simulink model "Train20"  (R2020b)
settings: Solver=VariableStepAuto  StartTime=0.0  StopTime=10.0  RelTol=1e-3
model workspace (MAT data in the model file):
  M_1 = 1
  M_10 = 1
  M_11 = 1
  M_12 = 1
  M_13 = 1
  M_14 = 1
  M_15 = 1
  M_16 = 1
  M_17 = 1
  M_18 = 1
  M_19 = 1
  M_2 = 1
  M_20 = 1
  M_3 = 1
  M_4 = 1
  M_5 = 1
  M_6 = 1
  M_7 = 1
  M_8 = 1
  M_9 = 1
  X0_10 = 1
  X0_11 = 1
  X0_12 = 1
  X0_13 = 1
  X0_14 = 1
  X0_15 = 1
  X0_16 = 1
  X0_17 = 1
  X0_18 = 1
  X0_19 = 1
  X0_2 = 1
  X0_20 = 1
  X0_3 = 1
  X0_4 = 1
  X0_5 = 1
  X0_6 = 1
  X0_7 = 1
  X0_8 = 1
  X0_9 = 1
  c = 8
  h = 1
  hs = 1
  k = 0.1
settings Model: Creator=zhenya  LastModifiedBy=zhenya

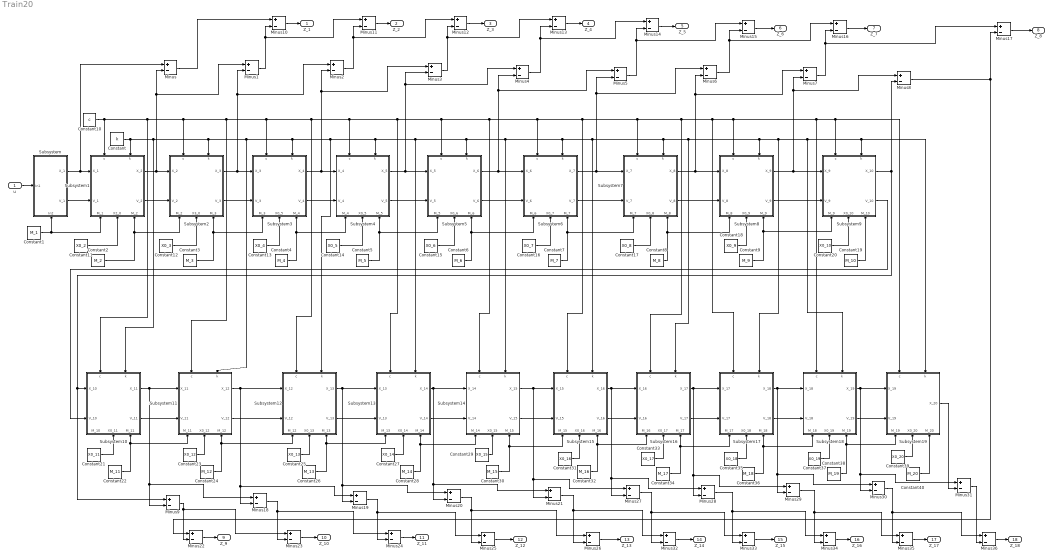
== system Train20 ==
  u : Inport
  Constant : Constant  Value=k
  Constant1 : Constant  Value=M_1
  Constant10 : Constant  Value=c
  Constant11 : Constant  Value=X0_2
  Constant12 : Constant  Value=X0_3
  Constant13 : Constant  Value=X0_4
  Constant14 : Constant  Value=X0_5
  Constant15 : Constant  Value=X0_6
  Constant16 : Constant  Value=X0_7
  Constant17 : Constant  Value=X0_8
  Constant18 : Constant  Value=X0_9
  Constant19 : Constant  Value=M_10
  Constant2 : Constant  Value=M_2
  Constant20 : Constant  Value=X0_10
  Constant21 : Constant  Value=X0_11
  Constant22 : Constant  Value=M_11
  Constant23 : Constant  Value=X0_12
  Constant24 : Constant  Value=M_12
  Constant25 : Constant  Value=X0_13
  Constant26 : Constant  Value=M_13
  Constant27 : Constant  Value=X0_14
  Constant28 : Constant  Value=M_14
  Constant29 : Constant  Value=X0_15
  Constant3 : Constant  Value=M_3
  Constant30 : Constant  Value=M_15
  Constant31 : Constant  Value=X0_16
  Constant32 : Constant  Value=M_16
  Constant33 : Constant  Value=X0_17
  Constant34 : Constant  Value=M_17
  Constant35 : Constant  Value=X0_18
  Constant36 : Constant  Value=M_18
  Constant37 : Constant  Value=X0_19
  Constant38 : Constant  Value=M_19
  Constant39 : Constant  Value=X0_20
  Constant4 : Constant  Value=M_4
  Constant40 : Constant  Value=M_20
  Constant5 : Constant  Value=M_5
  Constant6 : Constant  Value=M_6
  Constant7 : Constant  Value=M_7
  Constant8 : Constant  Value=M_8
  Constant9 : Constant  Value=M_9
  Minus{,1..36} (37 alike) : Sum  Inputs=+-
  Subsystem : Subsystem
      settings: PortSchema="{\"entries\":[{\"content\":{\"sides\":[{\"content\":{\"connectorIds\":[\"In1\"]},\"type\":\"ConnectorPlacement.EquallySpacedRectSide\",\"uuid\":\"34ca8425-fccb-4da0-be07-954015c86f74\"},{\"content\":{\"connectorIds\":[\"Out1\",\"Out2\"],\"side\":\"RIGHT\"},\"type\":\"ConnectorPlacement.EquallySpacedRectSide\",\"uuid\":\"a4a70c44-d99b-4f2f-bcd7-1dd85156dc1f\"},{\"content\":{\"connectorIds\":[],\"side\":\"TOP\"},\"type\":\"ConnectorPlacement.EquallySpacedRectSide\",\"uuid\":\"14968497-3b66-4f95-885e-db1a1d92cb6f\"},{\"content\":{\"connectorIds\":[\"In2\"],\"side\":\"BOTTOM\"},\"type\":\"ConnectorPlacement.EquallySpacedRectSide\",\"uuid\":\"7000d41a-f478-4b38-bf4d-e27f7f915c37\"},{\"content\":{\"connectorIds\":[],\"side\":\"HIDDEN\"},\"type\":\"ConnectorPlacement.EquallySpacedRectSide\",\"uuid\":\"79f1d2cd-3fc8-42f6-ae8b-07eaf6f97827\"}]},\"type\":\"ConnectorPlacement.EquallySpacedConnector\",\"uuid\":\"0ff0aa4c-6fa5-4dba-bb7c-396d165f33e0\"}],\"packageUris\":[\"http://schema.mathworks.com/mf0/Connector/R2020b\"],\"version\":\"1.0\"}"
  Subsystem1 : Subsystem
      settings: PortSchema="{\"entries\":[{\"content\":{\"sides\":[{\"content\":{\"connectorIds\":[\"In1\",\"In2\"]},\"type\":\"ConnectorPlacement.EquallySpacedRectSide\",\"uuid\":\"638557b6-12c9-401f-951d-5f98dd7903cc\"},{\"content\":{\"connectorIds\":[\"Out1\",\"Out2\"],\"side\":\"RIGHT\"},\"type\":\"ConnectorPlacement.EquallySpacedRectSide\",\"uuid\":\"d2d0712b-4eed-449a-bee8-cfe81cb0f76e\"},{\"content\":{\"connectorIds\":[\"In3\",\"In4\"],\"side\":\"TOP\"},\"type\":\"ConnectorPlacement.EquallySpacedRectSide\",\"uuid\":\"1558c73d-fb4f-4eb2-a0a5-81154d1cf643\"},{\"content\":{\"connectorIds\":[\"In5\",\"In6\",\"In7\"],\"side\":\"BOTTOM\"},\"type\":\"ConnectorPlacement.EquallySpacedRectSide\",\"uuid\":\"3af12584-476c-4d41-9154-a12458e629fd\"},{\"content\":{\"connectorIds\":[],\"side\":\"HIDDEN\"},\"type\":\"ConnectorPlacement.EquallySpacedRectSide\",\"uuid\":\"cdf596f7-1fd7-4460-9128-df53dc6c9dd6\"}]},\"type\":\"ConnectorPlacement.EquallySpacedConnector\",\"uuid\":\"66e3da69-735a-4605-b465-2e84808dff46\"}],\"packageUris\":[\"http://schema.mathworks.com/mf0/Connector/R2020b\"],\"version\":\"1.0\"}"
  Subsystem10 : Subsystem
      settings: PortSchema="{\"entries\":[{\"content\":{\"sides\":[{\"content\":{\"connectorIds\":[\"In1\",\"In2\"]},\"type\":\"ConnectorPlacement.EquallySpacedRectSide\",\"uuid\":\"638557b6-12c9-401f-951d-5f98dd7903cc\"},{\"content\":{\"connectorIds\":[\"Out1\",\"Out2\"],\"side\":\"RIGHT\"},\"type\":\"ConnectorPlacement.EquallySpacedRectSide\",\"uuid\":\"d2d0712b-4eed-449a-bee8-cfe81cb0f76e\"},{\"content\":{\"connectorIds\":[\"In3\",\"In4\"],\"side\":\"TOP\"},\"type\":\"ConnectorPlacement.EquallySpacedRectSide\",\"uuid\":\"1558c73d-fb4f-4eb2-a0a5-81154d1cf643\"},{\"content\":{\"connectorIds\":[\"In5\",\"In6\",\"In7\"],\"side\":\"BOTTOM\"},\"type\":\"ConnectorPlacement.EquallySpacedRectSide\",\"uuid\":\"3af12584-476c-4d41-9154-a12458e629fd\"},{\"content\":{\"connectorIds\":[],\"side\":\"HIDDEN\"},\"type\":\"ConnectorPlacement.EquallySpacedRectSide\",\"uuid\":\"cdf596f7-1fd7-4460-9128-df53dc6c9dd6\"}]},\"type\":\"ConnectorPlacement.EquallySpacedConnector\",\"uuid\":\"66e3da69-735a-4605-b465-2e84808dff46\"}],\"packageUris\":[\"http://schema.mathworks.com/mf0/Connector/R2020b\"],\"version\":\"1.0\"}"
  Subsystem11 : Subsystem
      settings: PortSchema="{\"entries\":[{\"content\":{\"sides\":[{\"content\":{\"connectorIds\":[\"In1\",\"In2\"]},\"type\":\"ConnectorPlacement.EquallySpacedRectSide\",\"uuid\":\"638557b6-12c9-401f-951d-5f98dd7903cc\"},{\"content\":{\"connectorIds\":[\"Out1\",\"Out2\"],\"side\":\"RIGHT\"},\"type\":\"ConnectorPlacement.EquallySpacedRectSide\",\"uuid\":\"d2d0712b-4eed-449a-bee8-cfe81cb0f76e\"},{\"content\":{\"connectorIds\":[\"In3\",\"In4\"],\"side\":\"TOP\"},\"type\":\"ConnectorPlacement.EquallySpacedRectSide\",\"uuid\":\"1558c73d-fb4f-4eb2-a0a5-81154d1cf643\"},{\"content\":{\"connectorIds\":[\"In5\",\"In6\",\"In7\"],\"side\":\"BOTTOM\"},\"type\":\"ConnectorPlacement.EquallySpacedRectSide\",\"uuid\":\"3af12584-476c-4d41-9154-a12458e629fd\"},{\"content\":{\"connectorIds\":[],\"side\":\"HIDDEN\"},\"type\":\"ConnectorPlacement.EquallySpacedRectSide\",\"uuid\":\"cdf596f7-1fd7-4460-9128-df53dc6c9dd6\"}]},\"type\":\"ConnectorPlacement.EquallySpacedConnector\",\"uuid\":\"66e3da69-735a-4605-b465-2e84808dff46\"}],\"packageUris\":[\"http://schema.mathworks.com/mf0/Connector/R2020b\"],\"version\":\"1.0\"}"
  Subsystem12 : Subsystem
      settings: PortSchema="{\"entries\":[{\"content\":{\"sides\":[{\"content\":{\"connectorIds\":[\"In1\",\"In2\"]},\"type\":\"ConnectorPlacement.EquallySpacedRectSide\",\"uuid\":\"638557b6-12c9-401f-951d-5f98dd7903cc\"},{\"content\":{\"connectorIds\":[\"Out1\",\"Out2\"],\"side\":\"RIGHT\"},\"type\":\"ConnectorPlacement.EquallySpacedRectSide\",\"uuid\":\"d2d0712b-4eed-449a-bee8-cfe81cb0f76e\"},{\"content\":{\"connectorIds\":[\"In3\",\"In4\"],\"side\":\"TOP\"},\"type\":\"ConnectorPlacement.EquallySpacedRectSide\",\"uuid\":\"1558c73d-fb4f-4eb2-a0a5-81154d1cf643\"},{\"content\":{\"connectorIds\":[\"In5\",\"In6\",\"In7\"],\"side\":\"BOTTOM\"},\"type\":\"ConnectorPlacement.EquallySpacedRectSide\",\"uuid\":\"3af12584-476c-4d41-9154-a12458e629fd\"},{\"content\":{\"connectorIds\":[],\"side\":\"HIDDEN\"},\"type\":\"ConnectorPlacement.EquallySpacedRectSide\",\"uuid\":\"cdf596f7-1fd7-4460-9128-df53dc6c9dd6\"}]},\"type\":\"ConnectorPlacement.EquallySpacedConnector\",\"uuid\":\"66e3da69-735a-4605-b465-2e84808dff46\"}],\"packageUris\":[\"http://schema.mathworks.com/mf0/Connector/R2020b\"],\"version\":\"1.0\"}"
  Subsystem13 : Subsystem
      settings: PortSchema="{\"entries\":[{\"content\":{\"sides\":[{\"content\":{\"connectorIds\":[\"In1\",\"In2\"]},\"type\":\"ConnectorPlacement.EquallySpacedRectSide\",\"uuid\":\"638557b6-12c9-401f-951d-5f98dd7903cc\"},{\"content\":{\"connectorIds\":[\"Out1\",\"Out2\"],\"side\":\"RIGHT\"},\"type\":\"ConnectorPlacement.EquallySpacedRectSide\",\"uuid\":\"d2d0712b-4eed-449a-bee8-cfe81cb0f76e\"},{\"content\":{\"connectorIds\":[\"In3\",\"In4\"],\"side\":\"TOP\"},\"type\":\"ConnectorPlacement.EquallySpacedRectSide\",\"uuid\":\"1558c73d-fb4f-4eb2-a0a5-81154d1cf643\"},{\"content\":{\"connectorIds\":[\"In5\",\"In6\",\"In7\"],\"side\":\"BOTTOM\"},\"type\":\"ConnectorPlacement.EquallySpacedRectSide\",\"uuid\":\"3af12584-476c-4d41-9154-a12458e629fd\"},{\"content\":{\"connectorIds\":[],\"side\":\"HIDDEN\"},\"type\":\"ConnectorPlacement.EquallySpacedRectSide\",\"uuid\":\"cdf596f7-1fd7-4460-9128-df53dc6c9dd6\"}]},\"type\":\"ConnectorPlacement.EquallySpacedConnector\",\"uuid\":\"66e3da69-735a-4605-b465-2e84808dff46\"}],\"packageUris\":[\"http://schema.mathworks.com/mf0/Connector/R2020b\"],\"version\":\"1.0\"}"
  Subsystem14 : Subsystem
      settings: PortSchema="{\"entries\":[{\"content\":{\"sides\":[{\"content\":{\"connectorIds\":[\"In1\",\"In2\"]},\"type\":\"ConnectorPlacement.EquallySpacedRectSide\",\"uuid\":\"638557b6-12c9-401f-951d-5f98dd7903cc\"},{\"content\":{\"connectorIds\":[\"Out1\",\"Out2\"],\"side\":\"RIGHT\"},\"type\":\"ConnectorPlacement.EquallySpacedRectSide\",\"uuid\":\"d2d0712b-4eed-449a-bee8-cfe81cb0f76e\"},{\"content\":{\"connectorIds\":[\"In3\",\"In4\"],\"side\":\"TOP\"},\"type\":\"ConnectorPlacement.EquallySpacedRectSide\",\"uuid\":\"1558c73d-fb4f-4eb2-a0a5-81154d1cf643\"},{\"content\":{\"connectorIds\":[\"In5\",\"In6\",\"In7\"],\"side\":\"BOTTOM\"},\"type\":\"ConnectorPlacement.EquallySpacedRectSide\",\"uuid\":\"3af12584-476c-4d41-9154-a12458e629fd\"},{\"content\":{\"connectorIds\":[],\"side\":\"HIDDEN\"},\"type\":\"ConnectorPlacement.EquallySpacedRectSide\",\"uuid\":\"cdf596f7-1fd7-4460-9128-df53dc6c9dd6\"}]},\"type\":\"ConnectorPlacement.EquallySpacedConnector\",\"uuid\":\"66e3da69-735a-4605-b465-2e84808dff46\"}],\"packageUris\":[\"http://schema.mathworks.com/mf0/Connector/R2020b\"],\"version\":\"1.0\"}"
  Subsystem15 : Subsystem
      settings: PortSchema="{\"entries\":[{\"content\":{\"sides\":[{\"content\":{\"connectorIds\":[\"In1\",\"In2\"]},\"type\":\"ConnectorPlacement.EquallySpacedRectSide\",\"uuid\":\"638557b6-12c9-401f-951d-5f98dd7903cc\"},{\"content\":{\"connectorIds\":[\"Out1\",\"Out2\"],\"side\":\"RIGHT\"},\"type\":\"ConnectorPlacement.EquallySpacedRectSide\",\"uuid\":\"d2d0712b-4eed-449a-bee8-cfe81cb0f76e\"},{\"content\":{\"connectorIds\":[\"In3\",\"In4\"],\"side\":\"TOP\"},\"type\":\"ConnectorPlacement.EquallySpacedRectSide\",\"uuid\":\"1558c73d-fb4f-4eb2-a0a5-81154d1cf643\"},{\"content\":{\"connectorIds\":[\"In5\",\"In6\",\"In7\"],\"side\":\"BOTTOM\"},\"type\":\"ConnectorPlacement.EquallySpacedRectSide\",\"uuid\":\"3af12584-476c-4d41-9154-a12458e629fd\"},{\"content\":{\"connectorIds\":[],\"side\":\"HIDDEN\"},\"type\":\"ConnectorPlacement.EquallySpacedRectSide\",\"uuid\":\"cdf596f7-1fd7-4460-9128-df53dc6c9dd6\"}]},\"type\":\"ConnectorPlacement.EquallySpacedConnector\",\"uuid\":\"66e3da69-735a-4605-b465-2e84808dff46\"}],\"packageUris\":[\"http://schema.mathworks.com/mf0/Connector/R2020b\"],\"version\":\"1.0\"}"
  Subsystem16 : Subsystem
      settings: PortSchema="{\"entries\":[{\"content\":{\"sides\":[{\"content\":{\"connectorIds\":[\"In1\",\"In2\"]},\"type\":\"ConnectorPlacement.EquallySpacedRectSide\",\"uuid\":\"638557b6-12c9-401f-951d-5f98dd7903cc\"},{\"content\":{\"connectorIds\":[\"Out1\",\"Out2\"],\"side\":\"RIGHT\"},\"type\":\"ConnectorPlacement.EquallySpacedRectSide\",\"uuid\":\"d2d0712b-4eed-449a-bee8-cfe81cb0f76e\"},{\"content\":{\"connectorIds\":[\"In3\",\"In4\"],\"side\":\"TOP\"},\"type\":\"ConnectorPlacement.EquallySpacedRectSide\",\"uuid\":\"1558c73d-fb4f-4eb2-a0a5-81154d1cf643\"},{\"content\":{\"connectorIds\":[\"In5\",\"In6\",\"In7\"],\"side\":\"BOTTOM\"},\"type\":\"ConnectorPlacement.EquallySpacedRectSide\",\"uuid\":\"3af12584-476c-4d41-9154-a12458e629fd\"},{\"content\":{\"connectorIds\":[],\"side\":\"HIDDEN\"},\"type\":\"ConnectorPlacement.EquallySpacedRectSide\",\"uuid\":\"cdf596f7-1fd7-4460-9128-df53dc6c9dd6\"}]},\"type\":\"ConnectorPlacement.EquallySpacedConnector\",\"uuid\":\"66e3da69-735a-4605-b465-2e84808dff46\"}],\"packageUris\":[\"http://schema.mathworks.com/mf0/Connector/R2020b\"],\"version\":\"1.0\"}"
  Subsystem17 : Subsystem
      settings: PortSchema="{\"entries\":[{\"content\":{\"sides\":[{\"content\":{\"connectorIds\":[\"In1\",\"In2\"]},\"type\":\"ConnectorPlacement.EquallySpacedRectSide\",\"uuid\":\"638557b6-12c9-401f-951d-5f98dd7903cc\"},{\"content\":{\"connectorIds\":[\"Out1\",\"Out2\"],\"side\":\"RIGHT\"},\"type\":\"ConnectorPlacement.EquallySpacedRectSide\",\"uuid\":\"d2d0712b-4eed-449a-bee8-cfe81cb0f76e\"},{\"content\":{\"connectorIds\":[\"In3\",\"In4\"],\"side\":\"TOP\"},\"type\":\"ConnectorPlacement.EquallySpacedRectSide\",\"uuid\":\"1558c73d-fb4f-4eb2-a0a5-81154d1cf643\"},{\"content\":{\"connectorIds\":[\"In5\",\"In6\",\"In7\"],\"side\":\"BOTTOM\"},\"type\":\"ConnectorPlacement.EquallySpacedRectSide\",\"uuid\":\"3af12584-476c-4d41-9154-a12458e629fd\"},{\"content\":{\"connectorIds\":[],\"side\":\"HIDDEN\"},\"type\":\"ConnectorPlacement.EquallySpacedRectSide\",\"uuid\":\"cdf596f7-1fd7-4460-9128-df53dc6c9dd6\"}]},\"type\":\"ConnectorPlacement.EquallySpacedConnector\",\"uuid\":\"66e3da69-735a-4605-b465-2e84808dff46\"}],\"packageUris\":[\"http://schema.mathworks.com/mf0/Connector/R2020b\"],\"version\":\"1.0\"}"
  Subsystem18 : Subsystem
      settings: PortSchema="{\"entries\":[{\"content\":{\"sides\":[{\"content\":{\"connectorIds\":[\"In1\",\"In2\"]},\"type\":\"ConnectorPlacement.EquallySpacedRectSide\",\"uuid\":\"638557b6-12c9-401f-951d-5f98dd7903cc\"},{\"content\":{\"connectorIds\":[\"Out1\",\"Out2\"],\"side\":\"RIGHT\"},\"type\":\"ConnectorPlacement.EquallySpacedRectSide\",\"uuid\":\"d2d0712b-4eed-449a-bee8-cfe81cb0f76e\"},{\"content\":{\"connectorIds\":[\"In3\",\"In4\"],\"side\":\"TOP\"},\"type\":\"ConnectorPlacement.EquallySpacedRectSide\",\"uuid\":\"1558c73d-fb4f-4eb2-a0a5-81154d1cf643\"},{\"content\":{\"connectorIds\":[\"In5\",\"In6\",\"In7\"],\"side\":\"BOTTOM\"},\"type\":\"ConnectorPlacement.EquallySpacedRectSide\",\"uuid\":\"3af12584-476c-4d41-9154-a12458e629fd\"},{\"content\":{\"connectorIds\":[],\"side\":\"HIDDEN\"},\"type\":\"ConnectorPlacement.EquallySpacedRectSide\",\"uuid\":\"cdf596f7-1fd7-4460-9128-df53dc6c9dd6\"}]},\"type\":\"ConnectorPlacement.EquallySpacedConnector\",\"uuid\":\"66e3da69-735a-4605-b465-2e84808dff46\"}],\"packageUris\":[\"http://schema.mathworks.com/mf0/Connector/R2020b\"],\"version\":\"1.0\"}"
  Subsystem19 : Subsystem
      settings: PortSchema="{\"entries\":[{\"content\":{\"sides\":[{\"content\":{\"connectorIds\":[\"In1\",\"In2\"]},\"type\":\"ConnectorPlacement.EquallySpacedRectSide\",\"uuid\":\"638557b6-12c9-401f-951d-5f98dd7903cc\"},{\"content\":{\"connectorIds\":[\"Out1\"],\"side\":\"RIGHT\"},\"type\":\"ConnectorPlacement.EquallySpacedRectSide\",\"uuid\":\"d2d0712b-4eed-449a-bee8-cfe81cb0f76e\"},{\"content\":{\"connectorIds\":[\"In3\",\"In4\"],\"side\":\"TOP\"},\"type\":\"ConnectorPlacement.EquallySpacedRectSide\",\"uuid\":\"1558c73d-fb4f-4eb2-a0a5-81154d1cf643\"},{\"content\":{\"connectorIds\":[\"In5\",\"In6\",\"In7\"],\"side\":\"BOTTOM\"},\"type\":\"ConnectorPlacement.EquallySpacedRectSide\",\"uuid\":\"3af12584-476c-4d41-9154-a12458e629fd\"},{\"content\":{\"connectorIds\":[],\"side\":\"HIDDEN\"},\"type\":\"ConnectorPlacement.EquallySpacedRectSide\",\"uuid\":\"cdf596f7-1fd7-4460-9128-df53dc6c9dd6\"}]},\"type\":\"ConnectorPlacement.EquallySpacedConnector\",\"uuid\":\"66e3da69-735a-4605-b465-2e84808dff46\"}],\"packageUris\":[\"http://schema.mathworks.com/mf0/Connector/R2020b\"],\"version\":\"1.0\"}"
  Subsystem2 : Subsystem
      settings: PortSchema="{\"entries\":[{\"content\":{\"sides\":[{\"content\":{\"connectorIds\":[\"In1\",\"In2\"]},\"type\":\"ConnectorPlacement.EquallySpacedRectSide\",\"uuid\":\"638557b6-12c9-401f-951d-5f98dd7903cc\"},{\"content\":{\"connectorIds\":[\"Out1\",\"Out2\"],\"side\":\"RIGHT\"},\"type\":\"ConnectorPlacement.EquallySpacedRectSide\",\"uuid\":\"d2d0712b-4eed-449a-bee8-cfe81cb0f76e\"},{\"content\":{\"connectorIds\":[\"In3\",\"In4\"],\"side\":\"TOP\"},\"type\":\"ConnectorPlacement.EquallySpacedRectSide\",\"uuid\":\"1558c73d-fb4f-4eb2-a0a5-81154d1cf643\"},{\"content\":{\"connectorIds\":[\"In5\",\"In6\",\"In7\"],\"side\":\"BOTTOM\"},\"type\":\"ConnectorPlacement.EquallySpacedRectSide\",\"uuid\":\"3af12584-476c-4d41-9154-a12458e629fd\"},{\"content\":{\"connectorIds\":[],\"side\":\"HIDDEN\"},\"type\":\"ConnectorPlacement.EquallySpacedRectSide\",\"uuid\":\"cdf596f7-1fd7-4460-9128-df53dc6c9dd6\"}]},\"type\":\"ConnectorPlacement.EquallySpacedConnector\",\"uuid\":\"66e3da69-735a-4605-b465-2e84808dff46\"}],\"packageUris\":[\"http://schema.mathworks.com/mf0/Connector/R2020b\"],\"version\":\"1.0\"}"
  Subsystem3 : Subsystem
      settings: PortSchema="{\"entries\":[{\"content\":{\"sides\":[{\"content\":{\"connectorIds\":[\"In1\",\"In2\"]},\"type\":\"ConnectorPlacement.EquallySpacedRectSide\",\"uuid\":\"638557b6-12c9-401f-951d-5f98dd7903cc\"},{\"content\":{\"connectorIds\":[\"Out1\",\"Out2\"],\"side\":\"RIGHT\"},\"type\":\"ConnectorPlacement.EquallySpacedRectSide\",\"uuid\":\"d2d0712b-4eed-449a-bee8-cfe81cb0f76e\"},{\"content\":{\"connectorIds\":[\"In3\",\"In4\"],\"side\":\"TOP\"},\"type\":\"ConnectorPlacement.EquallySpacedRectSide\",\"uuid\":\"1558c73d-fb4f-4eb2-a0a5-81154d1cf643\"},{\"content\":{\"connectorIds\":[\"In5\",\"In6\",\"In7\"],\"side\":\"BOTTOM\"},\"type\":\"ConnectorPlacement.EquallySpacedRectSide\",\"uuid\":\"3af12584-476c-4d41-9154-a12458e629fd\"},{\"content\":{\"connectorIds\":[],\"side\":\"HIDDEN\"},\"type\":\"ConnectorPlacement.EquallySpacedRectSide\",\"uuid\":\"cdf596f7-1fd7-4460-9128-df53dc6c9dd6\"}]},\"type\":\"ConnectorPlacement.EquallySpacedConnector\",\"uuid\":\"66e3da69-735a-4605-b465-2e84808dff46\"}],\"packageUris\":[\"http://schema.mathworks.com/mf0/Connector/R2020b\"],\"version\":\"1.0\"}"
  Subsystem4 : Subsystem
      settings: PortSchema="{\"entries\":[{\"content\":{\"sides\":[{\"content\":{\"connectorIds\":[\"In1\",\"In2\"]},\"type\":\"ConnectorPlacement.EquallySpacedRectSide\",\"uuid\":\"638557b6-12c9-401f-951d-5f98dd7903cc\"},{\"content\":{\"connectorIds\":[\"Out1\",\"Out2\"],\"side\":\"RIGHT\"},\"type\":\"ConnectorPlacement.EquallySpacedRectSide\",\"uuid\":\"d2d0712b-4eed-449a-bee8-cfe81cb0f76e\"},{\"content\":{\"connectorIds\":[\"In3\",\"In4\"],\"side\":\"TOP\"},\"type\":\"ConnectorPlacement.EquallySpacedRectSide\",\"uuid\":\"1558c73d-fb4f-4eb2-a0a5-81154d1cf643\"},{\"content\":{\"connectorIds\":[\"In5\",\"In6\",\"In7\"],\"side\":\"BOTTOM\"},\"type\":\"ConnectorPlacement.EquallySpacedRectSide\",\"uuid\":\"3af12584-476c-4d41-9154-a12458e629fd\"},{\"content\":{\"connectorIds\":[],\"side\":\"HIDDEN\"},\"type\":\"ConnectorPlacement.EquallySpacedRectSide\",\"uuid\":\"cdf596f7-1fd7-4460-9128-df53dc6c9dd6\"}]},\"type\":\"ConnectorPlacement.EquallySpacedConnector\",\"uuid\":\"66e3da69-735a-4605-b465-2e84808dff46\"}],\"packageUris\":[\"http://schema.mathworks.com/mf0/Connector/R2020b\"],\"version\":\"1.0\"}"
  Subsystem5 : Subsystem
      settings: PortSchema="{\"entries\":[{\"content\":{\"sides\":[{\"content\":{\"connectorIds\":[\"In1\",\"In2\"]},\"type\":\"ConnectorPlacement.EquallySpacedRectSide\",\"uuid\":\"638557b6-12c9-401f-951d-5f98dd7903cc\"},{\"content\":{\"connectorIds\":[\"Out1\",\"Out2\"],\"side\":\"RIGHT\"},\"type\":\"ConnectorPlacement.EquallySpacedRectSide\",\"uuid\":\"d2d0712b-4eed-449a-bee8-cfe81cb0f76e\"},{\"content\":{\"connectorIds\":[\"In3\",\"In4\"],\"side\":\"TOP\"},\"type\":\"ConnectorPlacement.EquallySpacedRectSide\",\"uuid\":\"1558c73d-fb4f-4eb2-a0a5-81154d1cf643\"},{\"content\":{\"connectorIds\":[\"In5\",\"In6\",\"In7\"],\"side\":\"BOTTOM\"},\"type\":\"ConnectorPlacement.EquallySpacedRectSide\",\"uuid\":\"3af12584-476c-4d41-9154-a12458e629fd\"},{\"content\":{\"connectorIds\":[],\"side\":\"HIDDEN\"},\"type\":\"ConnectorPlacement.EquallySpacedRectSide\",\"uuid\":\"cdf596f7-1fd7-4460-9128-df53dc6c9dd6\"}]},\"type\":\"ConnectorPlacement.EquallySpacedConnector\",\"uuid\":\"66e3da69-735a-4605-b465-2e84808dff46\"}],\"packageUris\":[\"http://schema.mathworks.com/mf0/Connector/R2020b\"],\"version\":\"1.0\"}"
  Subsystem6 : Subsystem
      settings: PortSchema="{\"entries\":[{\"content\":{\"sides\":[{\"content\":{\"connectorIds\":[\"In1\",\"In2\"]},\"type\":\"ConnectorPlacement.EquallySpacedRectSide\",\"uuid\":\"638557b6-12c9-401f-951d-5f98dd7903cc\"},{\"content\":{\"connectorIds\":[\"Out1\",\"Out2\"],\"side\":\"RIGHT\"},\"type\":\"ConnectorPlacement.EquallySpacedRectSide\",\"uuid\":\"d2d0712b-4eed-449a-bee8-cfe81cb0f76e\"},{\"content\":{\"connectorIds\":[\"In3\",\"In4\"],\"side\":\"TOP\"},\"type\":\"ConnectorPlacement.EquallySpacedRectSide\",\"uuid\":\"1558c73d-fb4f-4eb2-a0a5-81154d1cf643\"},{\"content\":{\"connectorIds\":[\"In5\",\"In6\",\"In7\"],\"side\":\"BOTTOM\"},\"type\":\"ConnectorPlacement.EquallySpacedRectSide\",\"uuid\":\"3af12584-476c-4d41-9154-a12458e629fd\"},{\"content\":{\"connectorIds\":[],\"side\":\"HIDDEN\"},\"type\":\"ConnectorPlacement.EquallySpacedRectSide\",\"uuid\":\"cdf596f7-1fd7-4460-9128-df53dc6c9dd6\"}]},\"type\":\"ConnectorPlacement.EquallySpacedConnector\",\"uuid\":\"66e3da69-735a-4605-b465-2e84808dff46\"}],\"packageUris\":[\"http://schema.mathworks.com/mf0/Connector/R2020b\"],\"version\":\"1.0\"}"
  Subsystem7 : Subsystem
      settings: PortSchema="{\"entries\":[{\"content\":{\"sides\":[{\"content\":{\"connectorIds\":[\"In1\",\"In2\"]},\"type\":\"ConnectorPlacement.EquallySpacedRectSide\",\"uuid\":\"638557b6-12c9-401f-951d-5f98dd7903cc\"},{\"content\":{\"connectorIds\":[\"Out1\",\"Out2\"],\"side\":\"RIGHT\"},\"type\":\"ConnectorPlacement.EquallySpacedRectSide\",\"uuid\":\"d2d0712b-4eed-449a-bee8-cfe81cb0f76e\"},{\"content\":{\"connectorIds\":[\"In3\",\"In4\"],\"side\":\"TOP\"},\"type\":\"ConnectorPlacement.EquallySpacedRectSide\",\"uuid\":\"1558c73d-fb4f-4eb2-a0a5-81154d1cf643\"},{\"content\":{\"connectorIds\":[\"In5\",\"In6\",\"In7\"],\"side\":\"BOTTOM\"},\"type\":\"ConnectorPlacement.EquallySpacedRectSide\",\"uuid\":\"3af12584-476c-4d41-9154-a12458e629fd\"},{\"content\":{\"connectorIds\":[],\"side\":\"HIDDEN\"},\"type\":\"ConnectorPlacement.EquallySpacedRectSide\",\"uuid\":\"cdf596f7-1fd7-4460-9128-df53dc6c9dd6\"}]},\"type\":\"ConnectorPlacement.EquallySpacedConnector\",\"uuid\":\"66e3da69-735a-4605-b465-2e84808dff46\"}],\"packageUris\":[\"http://schema.mathworks.com/mf0/Connector/R2020b\"],\"version\":\"1.0\"}"
  Subsystem8 : Subsystem
      settings: PortSchema="{\"entries\":[{\"content\":{\"sides\":[{\"content\":{\"connectorIds\":[\"In1\",\"In2\"]},\"type\":\"ConnectorPlacement.EquallySpacedRectSide\",\"uuid\":\"638557b6-12c9-401f-951d-5f98dd7903cc\"},{\"content\":{\"connectorIds\":[\"Out1\",\"Out2\"],\"side\":\"RIGHT\"},\"type\":\"ConnectorPlacement.EquallySpacedRectSide\",\"uuid\":\"d2d0712b-4eed-449a-bee8-cfe81cb0f76e\"},{\"content\":{\"connectorIds\":[\"In3\",\"In4\"],\"side\":\"TOP\"},\"type\":\"ConnectorPlacement.EquallySpacedRectSide\",\"uuid\":\"1558c73d-fb4f-4eb2-a0a5-81154d1cf643\"},{\"content\":{\"connectorIds\":[\"In5\",\"In6\",\"In7\"],\"side\":\"BOTTOM\"},\"type\":\"ConnectorPlacement.EquallySpacedRectSide\",\"uuid\":\"3af12584-476c-4d41-9154-a12458e629fd\"},{\"content\":{\"connectorIds\":[],\"side\":\"HIDDEN\"},\"type\":\"ConnectorPlacement.EquallySpacedRectSide\",\"uuid\":\"cdf596f7-1fd7-4460-9128-df53dc6c9dd6\"}]},\"type\":\"ConnectorPlacement.EquallySpacedConnector\",\"uuid\":\"66e3da69-735a-4605-b465-2e84808dff46\"}],\"packageUris\":[\"http://schema.mathworks.com/mf0/Connector/R2020b\"],\"version\":\"1.0\"}"
  Subsystem9 : Subsystem
      settings: PortSchema="{\"entries\":[{\"content\":{\"sides\":[{\"content\":{\"connectorIds\":[\"In1\",\"In2\"]},\"type\":\"ConnectorPlacement.EquallySpacedRectSide\",\"uuid\":\"638557b6-12c9-401f-951d-5f98dd7903cc\"},{\"content\":{\"connectorIds\":[\"Out1\",\"Out2\"],\"side\":\"RIGHT\"},\"type\":\"ConnectorPlacement.EquallySpacedRectSide\",\"uuid\":\"d2d0712b-4eed-449a-bee8-cfe81cb0f76e\"},{\"content\":{\"connectorIds\":[\"In3\",\"In4\"],\"side\":\"TOP\"},\"type\":\"ConnectorPlacement.EquallySpacedRectSide\",\"uuid\":\"1558c73d-fb4f-4eb2-a0a5-81154d1cf643\"},{\"content\":{\"connectorIds\":[\"In5\",\"In6\",\"In7\"],\"side\":\"BOTTOM\"},\"type\":\"ConnectorPlacement.EquallySpacedRectSide\",\"uuid\":\"3af12584-476c-4d41-9154-a12458e629fd\"},{\"content\":{\"connectorIds\":[],\"side\":\"HIDDEN\"},\"type\":\"ConnectorPlacement.EquallySpacedRectSide\",\"uuid\":\"cdf596f7-1fd7-4460-9128-df53dc6c9dd6\"}]},\"type\":\"ConnectorPlacement.EquallySpacedConnector\",\"uuid\":\"66e3da69-735a-4605-b465-2e84808dff46\"}],\"packageUris\":[\"http://schema.mathworks.com/mf0/Connector/R2020b\"],\"version\":\"1.0\"}"
  Z_1 : Outport
  Z_2 : Outport  Port=2
  Z_3 : Outport  Port=3
  Z_4 : Outport  Port=4
  Z_5 : Outport  Port=5
  Z_6 : Outport  Port=6
  Z_7 : Outport  Port=7
  Z_8 : Outport  Port=8
  Z_9 : Outport  Port=9
  Z_10 : Outport  Port=10
  Z_11 : Outport  Port=11
  Z_12 : Outport  Port=12
  Z_13 : Outport  Port=13
  Z_14 : Outport  Port=14
  Z_15 : Outport  Port=15
  Z_16 : Outport  Port=16
  Z_17 : Outport  Port=17
  Z_18 : Outport  Port=18
  wires:
  u/1 -> Subsystem/1(In1)
  Constant/1 -> Subsystem11/4(k), Subsystem12/4(k), Subsystem15/4(k), Subsystem17/4(k), Subsystem18/4(k), Subsystem19/4(k), Subsystem9/4(k), Subsystem8/4(k), Subsystem16/4(k), Subsystem7/4(k), Subsystem6/4(k), Subsystem14/4(k), Subsystem5/4(k), Subsystem13/4(k), Subsystem4/4(k), Subsystem3/4(k), Subsystem2/4(k), Subsystem10/4(k), Subsystem1/4(k)
  Constant2/1 -> Subsystem2/5(M_2), Subsystem1/7(M_2)
  Subsystem/2(V_1) -> Subsystem1/2(V_1)
  Constant10/1 -> Subsystem11/3(c), Subsystem12/3(c), Subsystem15/3(c), Subsystem16/3(c), Subsystem17/3(c), Subsystem18/3(c), Subsystem19/3(c), Subsystem9/3(c), Subsystem8/3(c), Subsystem7/3(c), Subsystem6/3(c), Subsystem14/3(c), Subsystem5/3(c), Subsystem13/3(c), Subsystem4/3(c), Subsystem3/3(c), Subsystem2/3(c), Subsystem10/3(c), Subsystem1/3(c)
  Constant1/1 -> Subsystem1/5(M_1), Subsystem/2(In2)
  Subsystem1/1(X_2) -> Minus1/1, Minus/2, Subsystem2/1(X_2)
  Subsystem1/2(V_2) -> Subsystem2/2(V_2)
  Constant3/1 -> Subsystem3/5(M_3), Subsystem2/7(M_3)
  Subsystem2/1(X_3) -> Minus2/1, Minus1/2, Subsystem3/1(X_3)
  Subsystem2/2(V_3) -> Subsystem3/2(V_3)
  Constant4/1 -> Subsystem4/5(M_4), Subsystem3/7(M_4)
  Subsystem3/2(V_4) -> Subsystem4/2(V_4)
  Subsystem3/1(X_4) -> Minus3/1, Minus2/2, Subsystem4/1(X_4)
  Constant5/1 -> Subsystem5/5(M_5), Subsystem4/7(M_5)
  Subsystem4/1(X_5) -> Minus4/1, Minus3/2, Subsystem5/1(X_5)
  Subsystem4/2(V_5) -> Subsystem5/2(V_5)
  Constant6/1 -> Subsystem6/5(M_6), Subsystem5/7(M_6)
  Subsystem5/1(X_6) -> Minus5/1, Minus4/2, Subsystem6/1(X_6)
  Subsystem5/2(V_6) -> Subsystem6/2(V_6)
  Constant7/1 -> Subsystem7/5(M_7), Subsystem6/7(M_7)
  Subsystem6/1(X_7) -> Minus6/1, Minus5/2, Subsystem7/1(X_7)
  Subsystem6/2(V_7) -> Subsystem7/2(V_7)
  Constant8/1 -> Subsystem8/5(M_8), Subsystem7/7(M_8)
  Subsystem7/1(X_8) -> Minus7/1, Minus6/2, Subsystem8/1(X_8)
  Subsystem7/2(V_8) -> Subsystem8/2(V_8)
  Constant9/1 -> Subsystem9/5(M_9), Subsystem8/7(M_9)
  Subsystem8/1(X_9) -> Subsystem9/1(X_9), Minus8/1, Minus7/2
  Subsystem/1(X_1) -> Minus/1, Subsystem1/1(X_1)
  Minus/1 -> Minus10/1
  Minus1/1 -> Minus11/1, Minus10/2
  Minus2/1 -> Minus12/1, Minus11/2
  Minus3/1 -> Minus13/1, Minus12/2
  Minus4/1 -> Minus14/1, Minus13/2
  Minus5/1 -> Minus15/1, Minus14/2
  Minus6/1 -> Minus16/1, Minus15/2
  Minus7/1 -> Minus16/2, Minus17/1
  Constant11/1 -> Subsystem1/6(X2_0)
  Constant12/1 -> Subsystem2/6(X3_0)
  Constant13/1 -> Subsystem3/6(X0_5)
  Constant14/1 -> Subsystem4/6(X0_5)
  Constant15/1 -> Subsystem5/6(X0_6)
  Constant16/1 -> Subsystem6/6(X0_7)
  Constant17/1 -> Subsystem7/6(X0_8)
  Constant18/1 -> Subsystem8/6(X0_9)
  Subsystem8/2(V_9) -> Subsystem9/2(V_9)
  Constant19/1 -> Subsystem9/7(M_10)
  Constant20/1 -> Subsystem9/6(X0_10)
  Subsystem9/1(X_10) -> Subsystem10/1(X_10), Minus9/1, Minus8/2
  Minus8/1 -> Minus17/2, Minus22/1
  Constant21/1 -> Subsystem10/6(X0_11)
  Constant22/1 -> Subsystem11/5(M_11), Subsystem10/7(M_11)
  Constant23/1 -> Subsystem11/6(X0_12)
  Constant24/1 -> Subsystem12/5(M_12), Subsystem11/7(M_12)
  Constant26/1 -> Subsystem13/5(M_13), Subsystem12/7(M_13)
  Constant25/1 -> Subsystem12/6(X0_13)
  Constant28/1 -> Subsystem14/5(M_14), Subsystem13/7(M_14)
  Constant27/1 -> Subsystem13/6(X0_14)
  Constant30/1 -> Subsystem15/5(M_15), Subsystem14/7(M_15)
  Constant29/1 -> Subsystem14/6(X0_15)
  Subsystem10/1(X_11) -> Minus18/1, Minus9/2, Subsystem11/1(X_11)
  Subsystem10/2(V_11) -> Subsystem11/2(V_11)
  Subsystem11/1(X_12) -> Minus19/1, Minus18/2, Subsystem12/1(X_12)
  Subsystem11/2(V_12) -> Subsystem12/2(V_12)
  Subsystem12/1(X_13) -> Minus20/1, Minus19/2, Subsystem13/1(X_13)
  Subsystem12/2(V_13) -> Subsystem13/2(V_13)
  Subsystem13/1(X_14) -> Minus21/1, Minus20/2, Subsystem14/1(X_14)
  Subsystem13/2(V_14) -> Subsystem14/2(V_14)
  Subsystem9/2(V_10) -> Subsystem10/2(V_10)
  Minus10/1 -> Z_1/1
  Minus11/1 -> Z_2/1
  Minus12/1 -> Z_3/1
  Minus13/1 -> Z_4/1
  Minus14/1 -> Z_5/1
  Minus15/1 -> Z_6/1
  Minus16/1 -> Z_7/1
  Minus17/1 -> Z_8/1
  Subsystem14/1(X_15) -> Subsystem15/1(X_15), Minus27/1, Minus21/2
  Minus9/1 -> Minus23/1, Minus22/2
  Minus22/1 -> Z_9/1
  Minus18/1 -> Minus24/1, Minus23/2
  Minus23/1 -> Z_10/1
  Minus19/1 -> Minus24/2, Minus25/1
  Minus24/1 -> Z_11/1
  Minus20/1 -> Minus26/1, Minus25/2
  Minus25/1 -> Z_12/1
  Minus21/1 -> Minus32/1, Minus26/2
  Minus26/1 -> Z_13/1
  Subsystem14/2(V_15) -> Subsystem15/2(V_15)
  Subsystem15/1(X_16) -> Minus28/1, Minus27/2, Subsystem16/1(X_16)
  Subsystem15/2(V_16) -> Subsystem16/2(V_16)
  Subsystem16/1(X_17) -> Minus29/1, Minus28/2, Subsystem17/1(X_17)
  Subsystem16/2(V_17) -> Subsystem17/2(V_17)
  Subsystem17/1(X_18) -> Minus30/1, Minus29/2, Subsystem18/1(X_18)
  Subsystem17/2(V_18) -> Subsystem18/2(V_18)
  Subsystem18/2(V_19) -> Subsystem19/2(V_19)
  Subsystem18/1(X_19) -> Minus31/1, Minus30/2, Subsystem19/1(X_19)
  Constant31/1 -> Subsystem15/6(X0_16)
  Constant32/1 -> Subsystem16/5(M_16), Subsystem15/7(M_16)
  Constant33/1 -> Subsystem16/6(X0_17)
  Constant34/1 -> Subsystem17/5(M_17), Subsystem16/7(M_17)
  Constant35/1 -> Subsystem17/6(X0_18)
  Constant36/1 -> Subsystem18/5(M_18), Subsystem17/7(M_18)
  Constant37/1 -> Subsystem18/6(X0_19)
  Constant38/1 -> Subsystem19/5(M_19), Subsystem18/7(M_19)
  Constant39/1 -> Subsystem19/6(X0_20)
  Constant40/1 -> Subsystem19/7(M_20)
  Subsystem19/1(X_20) -> Minus31/2
  Minus27/1 -> Minus33/1, Minus32/2
  Minus32/1 -> Z_14/1
  Minus28/1 -> Minus34/1, Minus33/2
  Minus33/1 -> Z_15/1
  Minus29/1 -> Minus35/1, Minus34/2
  Minus34/1 -> Z_16/1
  Minus30/1 -> Minus36/1, Minus35/2
  Minus35/1 -> Z_17/1
  Minus31/1 -> Minus36/2
  Minus36/1 -> Z_18/1

== system Train20/Subsystem ==
  In1 : Inport
  In2 : Inport  Port=2
  Divide : Product  Inputs=*/
  Integrator : Integrator
  Integrator2 : Integrator
  X_1 : Outport
  V_1 : Outport  Port=2
  wires:
  Integrator/1 -> X_1/1  "X_1"
  Integrator2/1 -> V_1/1, Integrator/1  "V_1"
  In1/1 -> Divide/1
  In2/1 -> Divide/2
  Divide/1 -> Integrator2/1

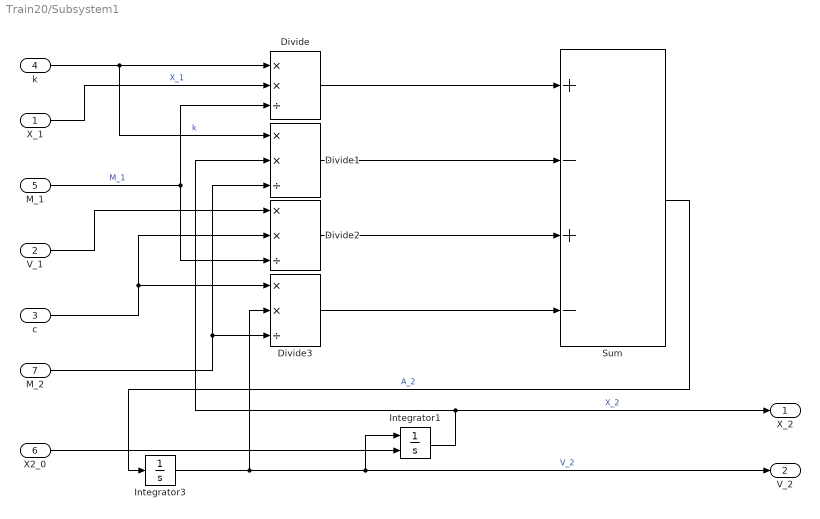
== system Train20/Subsystem1 ==
  X_1 : Inport
  V_1 : Inport  Port=2
  c : Inport  Port=3
  k : Inport  Port=4
  M_1 : Inport  Port=5
  X2_0 : Inport  Port=6
  M_2 : Inport  Port=7
  Divide{,1..3} (4 alike) : Product  Inputs=**/
  Integrator1 : Integrator  InitialConditionSource=external
  Integrator3 : Integrator
  Sum : Sum  Inputs=+-+-
  X_2 : Outport
  V_2 : Outport  Port=2
  wires:
  Divide2/1 -> Sum/3
  X_1/1 -> Divide/2  "X_1"
  Integrator3/1 -> Integrator1/1, V_2/1, Divide3/2  "V_2"
  Divide1/1 -> Sum/2
  V_1/1 -> Divide2/1
  Divide3/1 -> Sum/4
  Integrator1/1 -> Divide1/2, X_2/1  "X_2"
  Sum/1 -> Integrator3/1  "A_2"
  k/1 -> Divide1/1, Divide/1  "k"
  M_1/1 -> Divide2/3, Divide/3  "M_1"
  Divide/1 -> Sum/1
  M_2/1 -> Divide3/3, Divide1/3
  c/1 -> Divide2/2, Divide3/1
  X2_0/1 -> Integrator1/2

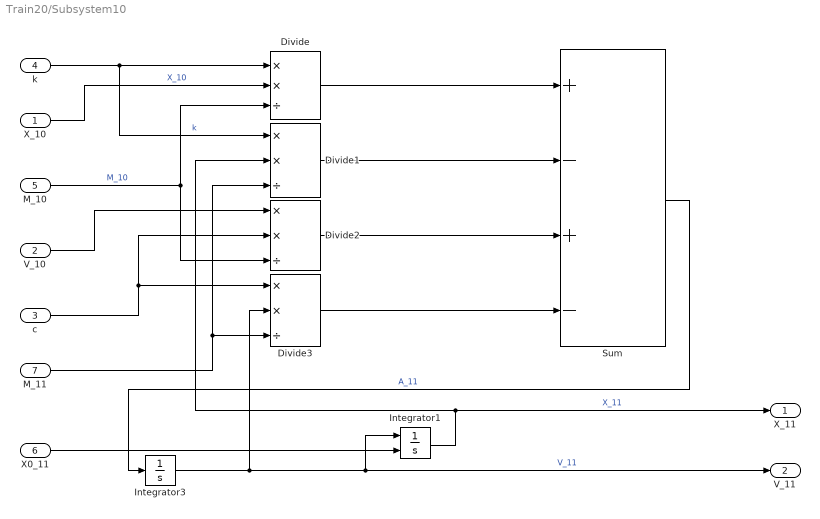
== system Train20/Subsystem10 ==
  X_10 : Inport
  V_10 : Inport  Port=2
  c : Inport  Port=3
  k : Inport  Port=4
  M_10 : Inport  Port=5
  X0_11 : Inport  Port=6
  M_11 : Inport  Port=7
  Divide{,1..3} (4 alike) : Product  Inputs=**/
  Integrator1 : Integrator  InitialConditionSource=external  InitialCondition=-62.5
  Integrator3 : Integrator
  Sum : Sum  Inputs=+-+-
  X_11 : Outport
  V_11 : Outport  Port=2
  wires:
  Divide2/1 -> Sum/3
  X_10/1 -> Divide/2  "X_10"
  Integrator3/1 -> Integrator1/1, V_11/1, Divide3/2  "V_11"
  Divide1/1 -> Sum/2
  V_10/1 -> Divide2/1
  Divide3/1 -> Sum/4
  Integrator1/1 -> Divide1/2, X_11/1  "X_11"
  Sum/1 -> Integrator3/1  "A_11"
  k/1 -> Divide1/1, Divide/1  "k"
  M_10/1 -> Divide2/3, Divide/3  "M_10"
  Divide/1 -> Sum/1
  M_11/1 -> Divide3/3, Divide1/3
  c/1 -> Divide2/2, Divide3/1
  X0_11/1 -> Integrator1/2

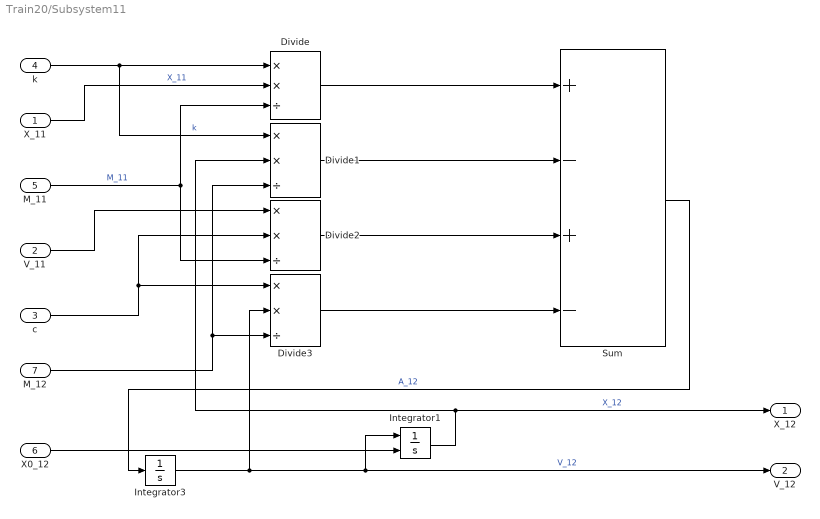
== system Train20/Subsystem11 ==
  X_11 : Inport
  V_11 : Inport  Port=2
  c : Inport  Port=3
  k : Inport  Port=4
  M_11 : Inport  Port=5
  X0_12 : Inport  Port=6
  M_12 : Inport  Port=7
  Divide{,1..3} (4 alike) : Product  Inputs=**/
  Integrator1 : Integrator  InitialConditionSource=external  InitialCondition=-72
  Integrator3 : Integrator
  Sum : Sum  Inputs=+-+-
  X_12 : Outport
  V_12 : Outport  Port=2
  wires:
  Divide2/1 -> Sum/3
  X_11/1 -> Divide/2  "X_11"
  Integrator3/1 -> Integrator1/1, V_12/1, Divide3/2  "V_12"
  Divide1/1 -> Sum/2
  V_11/1 -> Divide2/1
  Divide3/1 -> Sum/4
  Integrator1/1 -> Divide1/2, X_12/1  "X_12"
  Sum/1 -> Integrator3/1  "A_12"
  k/1 -> Divide1/1, Divide/1  "k"
  M_11/1 -> Divide2/3, Divide/3  "M_11"
  Divide/1 -> Sum/1
  M_12/1 -> Divide3/3, Divide1/3
  c/1 -> Divide2/2, Divide3/1
  X0_12/1 -> Integrator1/2

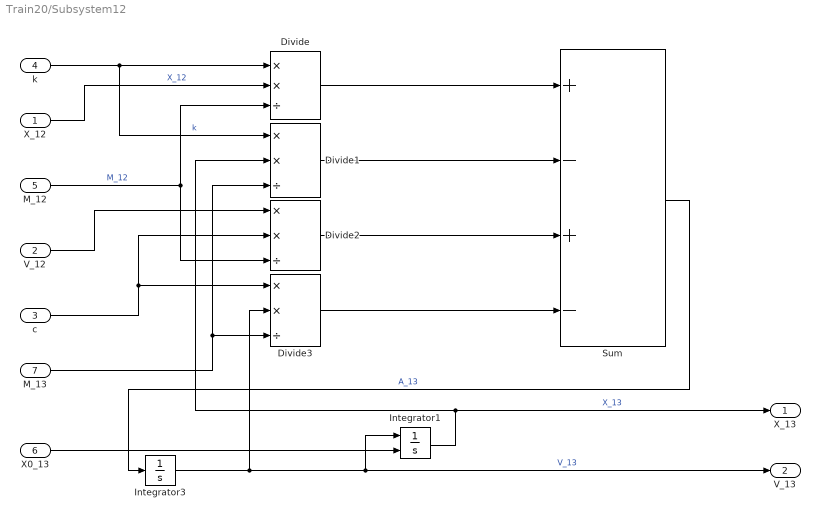
== system Train20/Subsystem12 ==
  X_12 : Inport
  V_12 : Inport  Port=2
  c : Inport  Port=3
  k : Inport  Port=4
  M_12 : Inport  Port=5
  X0_13 : Inport  Port=6
  M_13 : Inport  Port=7
  Divide{,1..3} (4 alike) : Product  Inputs=**/
  Integrator1 : Integrator  InitialConditionSource=external  InitialCondition=-80.5
  Integrator3 : Integrator
  Sum : Sum  Inputs=+-+-
  X_13 : Outport
  V_13 : Outport  Port=2
  wires:
  Divide2/1 -> Sum/3
  X_12/1 -> Divide/2  "X_12"
  Integrator3/1 -> Integrator1/1, V_13/1, Divide3/2  "V_13"
  Divide1/1 -> Sum/2
  V_12/1 -> Divide2/1
  Divide3/1 -> Sum/4
  Integrator1/1 -> Divide1/2, X_13/1  "X_13"
  Sum/1 -> Integrator3/1  "A_13"
  k/1 -> Divide1/1, Divide/1  "k"
  M_12/1 -> Divide2/3, Divide/3  "M_12"
  Divide/1 -> Sum/1
  M_13/1 -> Divide3/3, Divide1/3
  c/1 -> Divide2/2, Divide3/1
  X0_13/1 -> Integrator1/2

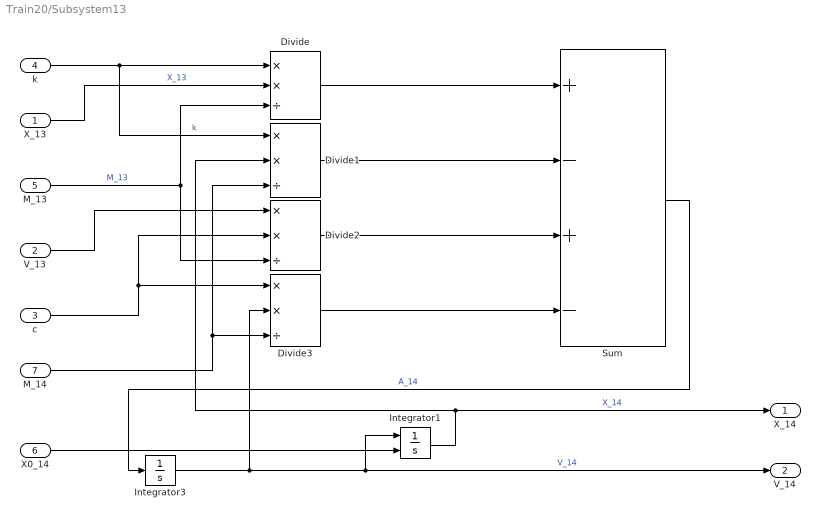
== system Train20/Subsystem13 ==
  X_13 : Inport
  V_13 : Inport  Port=2
  c : Inport  Port=3
  k : Inport  Port=4
  M_13 : Inport  Port=5
  X0_14 : Inport  Port=6
  M_14 : Inport  Port=7
  Divide{,1..3} (4 alike) : Product  Inputs=**/
  Integrator1 : Integrator  InitialConditionSource=external  InitialCondition=-88
  Integrator3 : Integrator
  Sum : Sum  Inputs=+-+-
  X_14 : Outport
  V_14 : Outport  Port=2
  wires:
  Divide2/1 -> Sum/3
  X_13/1 -> Divide/2  "X_13"
  Integrator3/1 -> V_14/1, Integrator1/1, Divide3/2  "V_14"
  Divide1/1 -> Sum/2
  V_13/1 -> Divide2/1
  Divide3/1 -> Sum/4
  Integrator1/1 -> Divide1/2, X_14/1  "X_14"
  Sum/1 -> Integrator3/1  "A_14"
  k/1 -> Divide1/1, Divide/1  "k"
  M_13/1 -> Divide2/3, Divide/3  "M_13"
  Divide/1 -> Sum/1
  M_14/1 -> Divide3/3, Divide1/3
  c/1 -> Divide2/2, Divide3/1
  X0_14/1 -> Integrator1/2

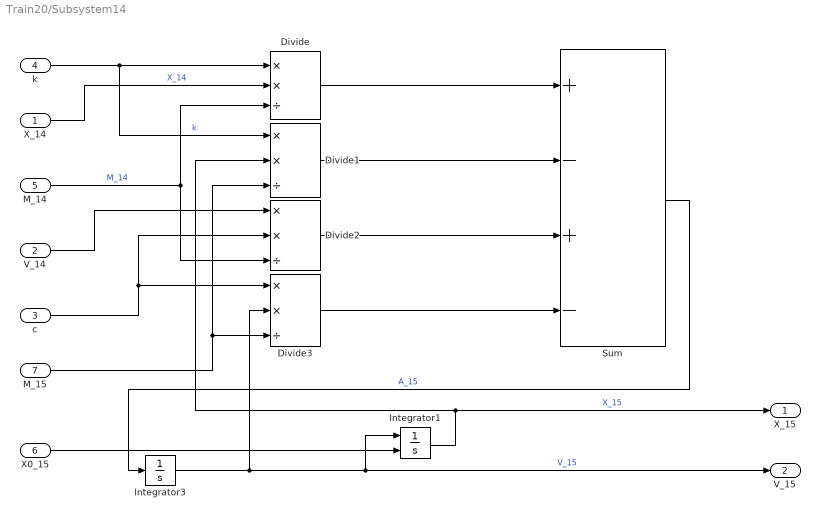
== system Train20/Subsystem14 ==
  X_14 : Inport
  V_14 : Inport  Port=2
  c : Inport  Port=3
  k : Inport  Port=4
  M_14 : Inport  Port=5
  X0_15 : Inport  Port=6
  M_15 : Inport  Port=7
  Divide{,1..3} (4 alike) : Product  Inputs=**/
  Integrator1 : Integrator  InitialConditionSource=external  InitialCondition=-88
  Integrator3 : Integrator
  Sum : Sum  Inputs=+-+-
  X_15 : Outport
  V_15 : Outport  Port=2
  wires:
  Divide2/1 -> Sum/3
  X_14/1 -> Divide/2  "X_14"
  Integrator3/1 -> Integrator1/1, V_15/1, Divide3/2  "V_15"
  Divide1/1 -> Sum/2
  V_14/1 -> Divide2/1
  Divide3/1 -> Sum/4
  Integrator1/1 -> Divide1/2, X_15/1  "X_15"
  Sum/1 -> Integrator3/1  "A_15"
  k/1 -> Divide1/1, Divide/1  "k"
  M_14/1 -> Divide2/3, Divide/3  "M_14"
  Divide/1 -> Sum/1
  M_15/1 -> Divide3/3, Divide1/3
  c/1 -> Divide2/2, Divide3/1
  X0_15/1 -> Integrator1/2

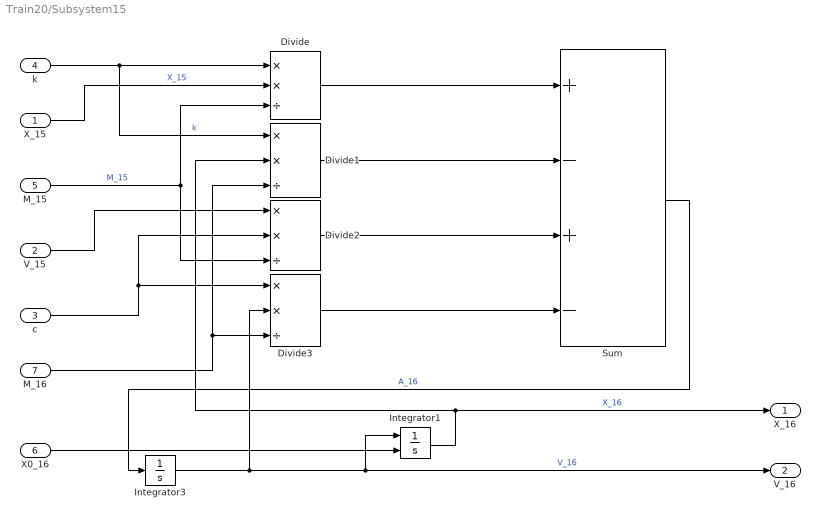
== system Train20/Subsystem15 ==
  X_15 : Inport
  V_15 : Inport  Port=2
  c : Inport  Port=3
  k : Inport  Port=4
  M_15 : Inport  Port=5
  X0_16 : Inport  Port=6
  M_16 : Inport  Port=7
  Divide{,1..3} (4 alike) : Product  Inputs=**/
  Integrator1 : Integrator  InitialConditionSource=external  InitialCondition=-62.5
  Integrator3 : Integrator
  Sum : Sum  Inputs=+-+-
  X_16 : Outport
  V_16 : Outport  Port=2
  wires:
  Divide2/1 -> Sum/3
  X_15/1 -> Divide/2  "X_15"
  Integrator3/1 -> Integrator1/1, V_16/1, Divide3/2  "V_16"
  Divide1/1 -> Sum/2
  V_15/1 -> Divide2/1
  Divide3/1 -> Sum/4
  Integrator1/1 -> Divide1/2, X_16/1  "X_16"
  Sum/1 -> Integrator3/1  "A_16"
  k/1 -> Divide1/1, Divide/1  "k"
  M_15/1 -> Divide2/3, Divide/3  "M_15"
  Divide/1 -> Sum/1
  M_16/1 -> Divide3/3, Divide1/3
  c/1 -> Divide2/2, Divide3/1
  X0_16/1 -> Integrator1/2

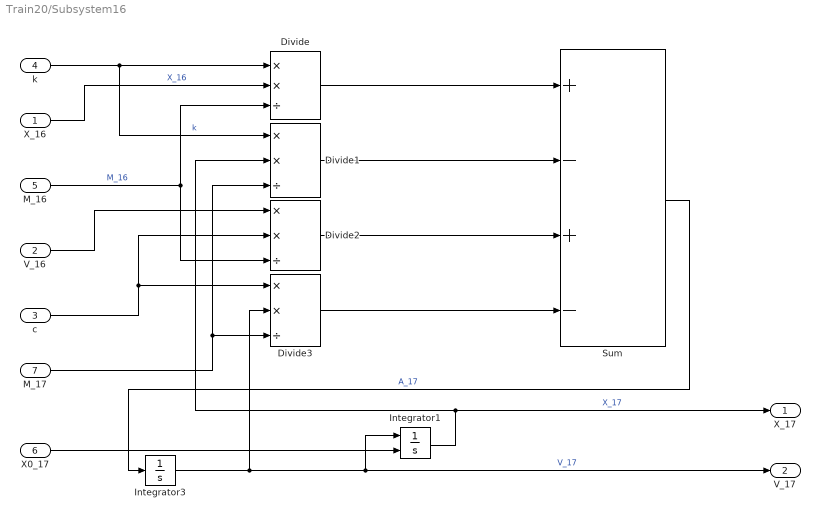
== system Train20/Subsystem16 ==
  X_16 : Inport
  V_16 : Inport  Port=2
  c : Inport  Port=3
  k : Inport  Port=4
  M_16 : Inport  Port=5
  X0_17 : Inport  Port=6
  M_17 : Inport  Port=7
  Divide{,1..3} (4 alike) : Product  Inputs=**/
  Integrator1 : Integrator  InitialConditionSource=external  InitialCondition=-72
  Integrator3 : Integrator
  Sum : Sum  Inputs=+-+-
  X_17 : Outport
  V_17 : Outport  Port=2
  wires:
  Divide2/1 -> Sum/3
  X_16/1 -> Divide/2  "X_16"
  Integrator3/1 -> Integrator1/1, V_17/1, Divide3/2  "V_17"
  Divide1/1 -> Sum/2
  V_16/1 -> Divide2/1
  Divide3/1 -> Sum/4
  Integrator1/1 -> Divide1/2, X_17/1  "X_17"
  Sum/1 -> Integrator3/1  "A_17"
  k/1 -> Divide1/1, Divide/1  "k"
  M_16/1 -> Divide2/3, Divide/3  "M_16"
  Divide/1 -> Sum/1
  M_17/1 -> Divide3/3, Divide1/3
  c/1 -> Divide2/2, Divide3/1
  X0_17/1 -> Integrator1/2

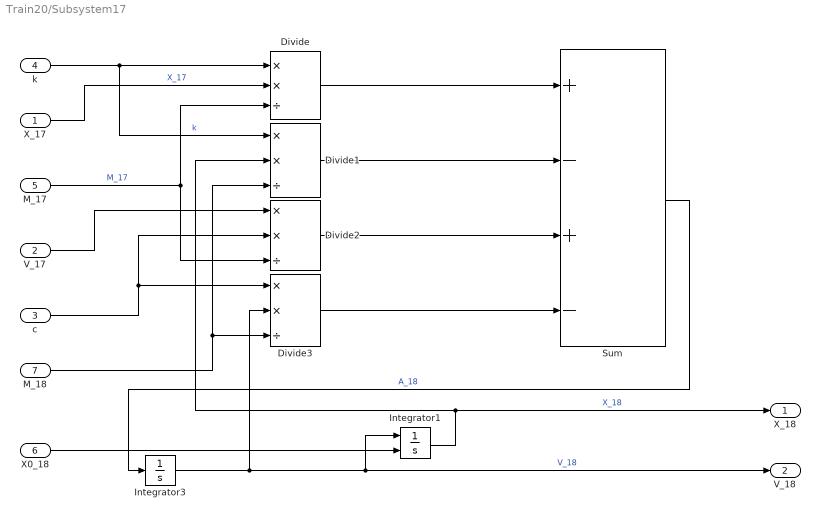
== system Train20/Subsystem17 ==
  X_17 : Inport
  V_17 : Inport  Port=2
  c : Inport  Port=3
  k : Inport  Port=4
  M_17 : Inport  Port=5
  X0_18 : Inport  Port=6
  M_18 : Inport  Port=7
  Divide{,1..3} (4 alike) : Product  Inputs=**/
  Integrator1 : Integrator  InitialConditionSource=external  InitialCondition=-80.5
  Integrator3 : Integrator
  Sum : Sum  Inputs=+-+-
  X_18 : Outport
  V_18 : Outport  Port=2
  wires:
  Divide2/1 -> Sum/3
  X_17/1 -> Divide/2  "X_17"
  Integrator3/1 -> Integrator1/1, V_18/1, Divide3/2  "V_18"
  Divide1/1 -> Sum/2
  V_17/1 -> Divide2/1
  Divide3/1 -> Sum/4
  Integrator1/1 -> Divide1/2, X_18/1  "X_18"
  Sum/1 -> Integrator3/1  "A_18"
  k/1 -> Divide1/1, Divide/1  "k"
  M_17/1 -> Divide2/3, Divide/3  "M_17"
  Divide/1 -> Sum/1
  M_18/1 -> Divide3/3, Divide1/3
  c/1 -> Divide2/2, Divide3/1
  X0_18/1 -> Integrator1/2

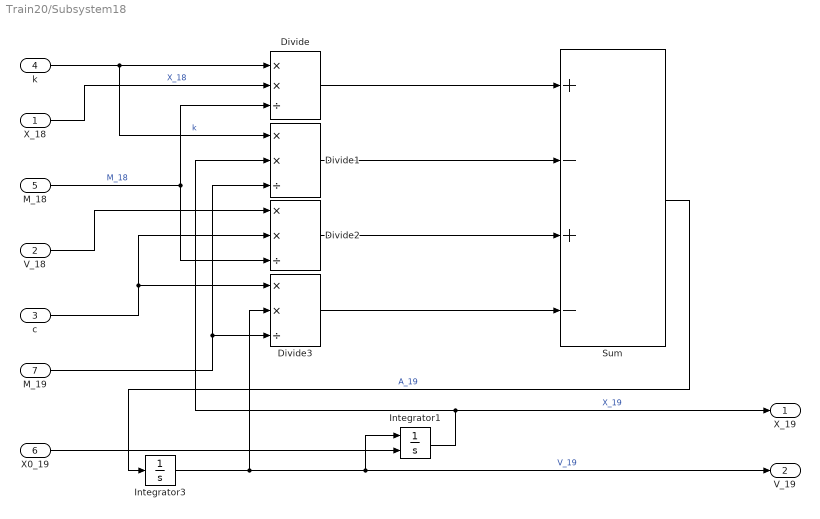
== system Train20/Subsystem18 ==
  X_18 : Inport
  V_18 : Inport  Port=2
  c : Inport  Port=3
  k : Inport  Port=4
  M_18 : Inport  Port=5
  X0_19 : Inport  Port=6
  M_19 : Inport  Port=7
  Divide{,1..3} (4 alike) : Product  Inputs=**/
  Integrator1 : Integrator  InitialConditionSource=external  InitialCondition=-88
  Integrator3 : Integrator
  Sum : Sum  Inputs=+-+-
  X_19 : Outport
  V_19 : Outport  Port=2
  wires:
  Divide2/1 -> Sum/3
  X_18/1 -> Divide/2  "X_18"
  Integrator3/1 -> V_19/1, Integrator1/1, Divide3/2  "V_19"
  Divide1/1 -> Sum/2
  V_18/1 -> Divide2/1
  Divide3/1 -> Sum/4
  Integrator1/1 -> Divide1/2, X_19/1  "X_19"
  Sum/1 -> Integrator3/1  "A_19"
  k/1 -> Divide1/1, Divide/1  "k"
  M_18/1 -> Divide2/3, Divide/3  "M_18"
  Divide/1 -> Sum/1
  M_19/1 -> Divide3/3, Divide1/3
  c/1 -> Divide2/2, Divide3/1
  X0_19/1 -> Integrator1/2

== system Train20/Subsystem19 ==
  X_19 : Inport
  V_19 : Inport  Port=2
  c : Inport  Port=3
  k : Inport  Port=4
  M_19 : Inport  Port=5
  X0_20 : Inport  Port=6
  M_20 : Inport  Port=7
  Divide{,1..3} (4 alike) : Product  Inputs=**/
  Integrator1 : Integrator  InitialConditionSource=external  InitialCondition=-88
  Integrator3 : Integrator
  Sum : Sum  Inputs=+-+-
  X_20 : Outport
  wires:
  Divide2/1 -> Sum/3
  X_19/1 -> Divide/2  "X_19"
  Integrator3/1 -> Integrator1/1, Divide3/2  "V_20"
  Divide1/1 -> Sum/2
  V_19/1 -> Divide2/1
  Divide3/1 -> Sum/4
  Integrator1/1 -> Divide1/2, X_20/1  "X_20"
  Sum/1 -> Integrator3/1  "A_20"
  k/1 -> Divide1/1, Divide/1  "k"
  M_19/1 -> Divide2/3, Divide/3  "M_19"
  Divide/1 -> Sum/1
  M_20/1 -> Divide3/3, Divide1/3
  c/1 -> Divide2/2, Divide3/1
  X0_20/1 -> Integrator1/2

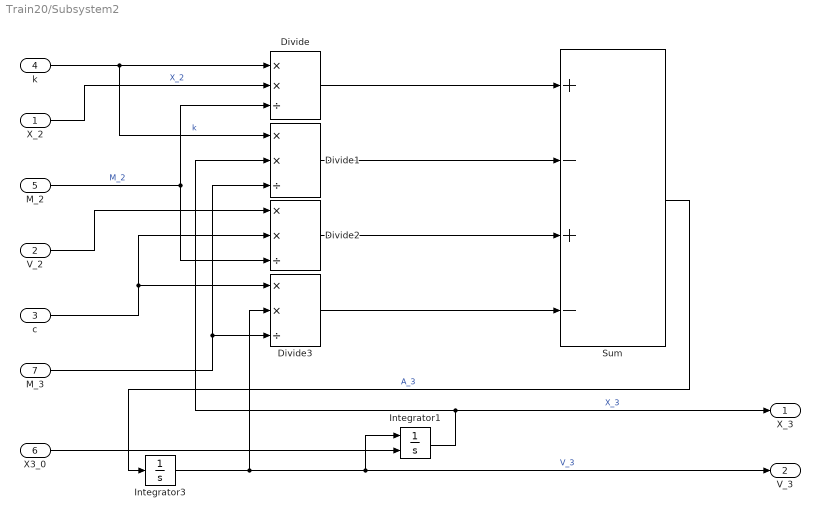
== system Train20/Subsystem2 ==
  X_2 : Inport
  V_2 : Inport  Port=2
  c : Inport  Port=3
  k : Inport  Port=4
  M_2 : Inport  Port=5
  X3_0 : Inport  Port=6
  M_3 : Inport  Port=7
  Divide{,1..3} (4 alike) : Product  Inputs=**/
  Integrator1 : Integrator  InitialConditionSource=external  InitialCondition=-28
  Integrator3 : Integrator
  Sum : Sum  Inputs=+-+-
  X_3 : Outport
  V_3 : Outport  Port=2
  wires:
  Divide2/1 -> Sum/3
  X_2/1 -> Divide/2  "X_2"
  Integrator3/1 -> Integrator1/1, V_3/1, Divide3/2  "V_3"
  Divide1/1 -> Sum/2
  V_2/1 -> Divide2/1
  Divide3/1 -> Sum/4
  Integrator1/1 -> Divide1/2, X_3/1  "X_3"
  Sum/1 -> Integrator3/1  "A_3"
  k/1 -> Divide1/1, Divide/1  "k"
  M_2/1 -> Divide2/3, Divide/3  "M_2"
  Divide/1 -> Sum/1
  M_3/1 -> Divide3/3, Divide1/3
  c/1 -> Divide2/2, Divide3/1
  X3_0/1 -> Integrator1/2

== system Train20/Subsystem3 ==
  X_3 : Inport
  V_3 : Inport  Port=2
  c : Inport  Port=3
  k : Inport  Port=4
  M_3 : Inport  Port=5
  X0_5 : Inport  Port=6
  M_4 : Inport  Port=7
  Divide{,1..3} (4 alike) : Product  Inputs=**/
  Integrator1 : Integrator  InitialConditionSource=external  InitialCondition=-40.5
  Integrator3 : Integrator
  Sum : Sum  Inputs=+-+-
  X_4 : Outport
  V_4 : Outport  Port=2
  wires:
  Divide2/1 -> Sum/3
  X_3/1 -> Divide/2  "X_3"
  Integrator3/1 -> Integrator1/1, V_4/1, Divide3/2  "V_4"
  Divide1/1 -> Sum/2
  V_3/1 -> Divide2/1
  Divide3/1 -> Sum/4
  Integrator1/1 -> Divide1/2, X_4/1  "X_4"
  Sum/1 -> Integrator3/1  "A_4"
  k/1 -> Divide1/1, Divide/1  "k"
  M_3/1 -> Divide2/3, Divide/3  "M_1"
  Divide/1 -> Sum/1
  M_4/1 -> Divide3/3, Divide1/3
  c/1 -> Divide2/2, Divide3/1
  X0_5/1 -> Integrator1/2

== system Train20/Subsystem4 ==
  X_4 : Inport
  V_4 : Inport  Port=2
  c : Inport  Port=3
  k : Inport  Port=4
  M_4 : Inport  Port=5
  X0_5 : Inport  Port=6
  M_5 : Inport  Port=7
  Divide{,1..3} (4 alike) : Product  Inputs=**/
  Integrator1 : Integrator  InitialConditionSource=external  InitialCondition=-52
  Integrator3 : Integrator
  Sum : Sum  Inputs=+-+-
  X_5 : Outport
  V_5 : Outport  Port=2
  wires:
  Divide2/1 -> Sum/3
  X_4/1 -> Divide/2  "X_4"
  Integrator3/1 -> Integrator1/1, V_5/1, Divide3/2  "V_5"
  Divide1/1 -> Sum/2
  V_4/1 -> Divide2/1
  Divide3/1 -> Sum/4
  Integrator1/1 -> Divide1/2, X_5/1  "X_5"
  Sum/1 -> Integrator3/1  "A_5"
  k/1 -> Divide1/1, Divide/1  "k"
  M_4/1 -> Divide2/3, Divide/3  "M_4"
  Divide/1 -> Sum/1
  M_5/1 -> Divide3/3, Divide1/3
  c/1 -> Divide2/2, Divide3/1
  X0_5/1 -> Integrator1/2

== system Train20/Subsystem5 ==
  X_5 : Inport
  V_5 : Inport  Port=2
  c : Inport  Port=3
  k : Inport  Port=4
  M_5 : Inport  Port=5
  X0_6 : Inport  Port=6
  M_6 : Inport  Port=7
  Divide{,1..3} (4 alike) : Product  Inputs=**/
  Integrator1 : Integrator  InitialConditionSource=external  InitialCondition=-62.5
  Integrator3 : Integrator
  Sum : Sum  Inputs=+-+-
  X_6 : Outport
  V_6 : Outport  Port=2
  wires:
  Divide2/1 -> Sum/3
  X_5/1 -> Divide/2  "X_5"
  Integrator3/1 -> Integrator1/1, V_6/1, Divide3/2  "V_6"
  Divide1/1 -> Sum/2
  V_5/1 -> Divide2/1
  Divide3/1 -> Sum/4
  Integrator1/1 -> Divide1/2, X_6/1  "X_6"
  Sum/1 -> Integrator3/1  "A_6"
  k/1 -> Divide1/1, Divide/1  "k"
  M_5/1 -> Divide2/3, Divide/3  "M_4"
  Divide/1 -> Sum/1
  M_6/1 -> Divide3/3, Divide1/3
  c/1 -> Divide2/2, Divide3/1
  X0_6/1 -> Integrator1/2

== system Train20/Subsystem6 ==
  X_6 : Inport
  V_6 : Inport  Port=2
  c : Inport  Port=3
  k : Inport  Port=4
  M_6 : Inport  Port=5
  X0_7 : Inport  Port=6
  M_7 : Inport  Port=7
  Divide{,1..3} (4 alike) : Product  Inputs=**/
  Integrator1 : Integrator  InitialConditionSource=external  InitialCondition=-72
  Integrator3 : Integrator
  Sum : Sum  Inputs=+-+-
  X_7 : Outport
  V_7 : Outport  Port=2
  wires:
  Divide2/1 -> Sum/3
  X_6/1 -> Divide/2  "X_6"
  Integrator3/1 -> Integrator1/1, V_7/1, Divide3/2  "V_7"
  Divide1/1 -> Sum/2
  V_6/1 -> Divide2/1
  Divide3/1 -> Sum/4
  Integrator1/1 -> Divide1/2, X_7/1  "X_7"
  Sum/1 -> Integrator3/1  "A_7"
  k/1 -> Divide1/1, Divide/1  "k"
  M_6/1 -> Divide2/3, Divide/3  "M_6"
  Divide/1 -> Sum/1
  M_7/1 -> Divide3/3, Divide1/3
  c/1 -> Divide2/2, Divide3/1
  X0_7/1 -> Integrator1/2

== system Train20/Subsystem7 ==
  X_7 : Inport
  V_7 : Inport  Port=2
  c : Inport  Port=3
  k : Inport  Port=4
  M_7 : Inport  Port=5
  X0_8 : Inport  Port=6
  M_8 : Inport  Port=7
  Divide{,1..3} (4 alike) : Product  Inputs=**/
  Integrator1 : Integrator  InitialConditionSource=external  InitialCondition=-80.5
  Integrator3 : Integrator
  Sum : Sum  Inputs=+-+-
  X_8 : Outport
  V_8 : Outport  Port=2
  wires:
  Divide2/1 -> Sum/3
  X_7/1 -> Divide/2  "X_7"
  Integrator3/1 -> Integrator1/1, V_8/1, Divide3/2  "V_8"
  Divide1/1 -> Sum/2
  V_7/1 -> Divide2/1
  Divide3/1 -> Sum/4
  Integrator1/1 -> Divide1/2, X_8/1  "X_8"
  Sum/1 -> Integrator3/1  "A_8"
  k/1 -> Divide1/1, Divide/1  "k"
  M_7/1 -> Divide2/3, Divide/3  "M_7"
  Divide/1 -> Sum/1
  M_8/1 -> Divide3/3, Divide1/3
  c/1 -> Divide2/2, Divide3/1
  X0_8/1 -> Integrator1/2

== system Train20/Subsystem8 ==
  X_8 : Inport
  V_8 : Inport  Port=2
  c : Inport  Port=3
  k : Inport  Port=4
  M_8 : Inport  Port=5
  X0_9 : Inport  Port=6
  M_9 : Inport  Port=7
  Divide{,1..3} (4 alike) : Product  Inputs=**/
  Integrator1 : Integrator  InitialConditionSource=external  InitialCondition=-88
  Integrator3 : Integrator
  Sum : Sum  Inputs=+-+-
  X_9 : Outport
  V_9 : Outport  Port=2
  wires:
  Divide2/1 -> Sum/3
  X_8/1 -> Divide/2  "X_8"
  Integrator3/1 -> V_9/1, Integrator1/1, Divide3/2  "V_9"
  Divide1/1 -> Sum/2
  V_8/1 -> Divide2/1
  Divide3/1 -> Sum/4
  Integrator1/1 -> Divide1/2, X_9/1  "X_9"
  Sum/1 -> Integrator3/1  "A_9"
  k/1 -> Divide1/1, Divide/1  "k"
  M_8/1 -> Divide2/3, Divide/3  "M_8"
  Divide/1 -> Sum/1
  M_9/1 -> Divide3/3, Divide1/3
  c/1 -> Divide2/2, Divide3/1
  X0_9/1 -> Integrator1/2

== system Train20/Subsystem9 ==
  X_9 : Inport
  V_9 : Inport  Port=2
  c : Inport  Port=3
  k : Inport  Port=4
  M_9 : Inport  Port=5
  X0_10 : Inport  Port=6
  M_10 : Inport  Port=7
  Divide{,1..3} (4 alike) : Product  Inputs=**/
  Integrator1 : Integrator  InitialConditionSource=external  InitialCondition=-88
  Integrator3 : Integrator
  Sum : Sum  Inputs=+-+-
  X_10 : Outport
  V_10 : Outport  Port=2
  wires:
  Divide2/1 -> Sum/3
  X_9/1 -> Divide/2  "X_9"
  Integrator3/1 -> Integrator1/1, V_10/1, Divide3/2  "V_10"
  Divide1/1 -> Sum/2
  V_9/1 -> Divide2/1
  Divide3/1 -> Sum/4
  Integrator1/1 -> Divide1/2, X_10/1  "X_10"
  Sum/1 -> Integrator3/1  "A_10"
  k/1 -> Divide1/1, Divide/1  "k"
  M_9/1 -> Divide2/3, Divide/3  "M_9"
  Divide/1 -> Sum/1
  M_10/1 -> Divide3/3, Divide1/3
  c/1 -> Divide2/2, Divide3/1
  X0_10/1 -> Integrator1/2
